simulink model "UAV_sync_unknown_gap_sim"  (R2018b)
settings: Solver=ode23tb  StartTime=0.0  StopTime=35  RelTol=1e-3
values from neighbouring files (symbols this model uses):
  Bm = [zeros(6,6); eye(6)]    [UAV_sync_unknown.m]    (also in UAV_sync_unknown_gap.m)
  C_rho = 1.225    [SC42120_UAV_Preconditions.m]
  D0 = [M0 0 0 0 0 0 ... (first row only)    [SC42120_UAV_Preconditions.m]
  Derivative_gain_phi = 50    [SC42120_UAV_Preconditions.m]
  Derivative_gain_psi = 50    [SC42120_UAV_Preconditions.m]
  Derivative_gain_theta = 50    [SC42120_UAV_Preconditions.m]
  Derivative_gain_x = 50    [SC42120_UAV_Preconditions.m]
  Derivative_gain_y = 50    [SC42120_UAV_Preconditions.m]
  Derivative_gain_z = 50    [SC42120_UAV_Preconditions.m]
  G = 9.80665    [SC42120_UAV_Preconditions.m]
  g0 = [0;0;-M0*G;0;0;0]    [SC42120_UAV_Preconditions.m]
  I0 = [0.02 0 -0.01 ... (first row only)    [SC42120_UAV_Preconditions.m]
  I2 = 2*[0.1 0 -0.01 ... (first row only)    [UAV_sync_known.m]    (also in UAV_sync_unknown.m; UAV_sync_unknown_gap.m)
  InitWind = [0;0;0]    [SC42120_UAV_Preconditions.m]
  Kp = diag(P)    [SC42120_UAV_Preconditions.m]
  Kv = diag(V)    [SC42120_UAV_Preconditions.m]
  M0 = 10    [SC42120_UAV_Preconditions.m]
  M1 = 20    [UAV_sync_known.m]    (also in UAV_sync_unknown.m; UAV_sync_unknown_gap.m)
  M2 = 30    [UAV_sync_known.m]    (also in UAV_sync_unknown.m; UAV_sync_unknown_gap.m)
  M3 = 40    [UAV_sync_known.m]    (also in UAV_sync_unknown.m; UAV_sync_unknown_gap.m)
  M4 = 50    [UAV_sync_known.m]    (also in UAV_sync_unknown.m; UAV_sync_unknown_gap.m)
  P = [Proportional_x Proportional_y Proportional_z Proportional_phi Proportional_theta Proportional_psi]    [SC42120_UAV_Preconditions.m]    (also in UAV_sync_unknown.m = lyap(Am',Q); UAV_sync_unknown_gap.m = lyap(Am',Q); drawDATCOMaircraft.m = temparray)
  Proportional_phi = 50    [SC42120_UAV_Preconditions.m]
  Proportional_psi = 50    [SC42120_UAV_Preconditions.m]
  Proportional_theta = 50    [SC42120_UAV_Preconditions.m]
  Proportional_x = 50    [SC42120_UAV_Preconditions.m]
  Proportional_y = 50    [SC42120_UAV_Preconditions.m]
  Proportional_z = 50    [SC42120_UAV_Preconditions.m]
  x_gap = 50    [UAV_sync_unknown_gap.m]
  y_gap = 100    [UAV_sync_unknown_gap.m]
undefined symbols (not defined in the file or in its folder): Aero, APlane, Bxl, C, Ctr, deg, DiscIntNeverNeededParam, F, Guid, Init, Light, MIL, Path, rad, s, Trim, Utility
libraries: aerolibconvert2 x37, sharedutil x20, simulink x15, dspsigops x7, shared6dof x6, aerolibasang x4, simulink_extras x3, aerolibadyn x1, aerolibtransform2 x1, aerolibwind2 x1
(part 1 of 7)
settings Model: Creator=kunal  LastModifiedBy=TUDelft SID
settings SolverCC: ZeroCrossAlgorithm=Adaptive

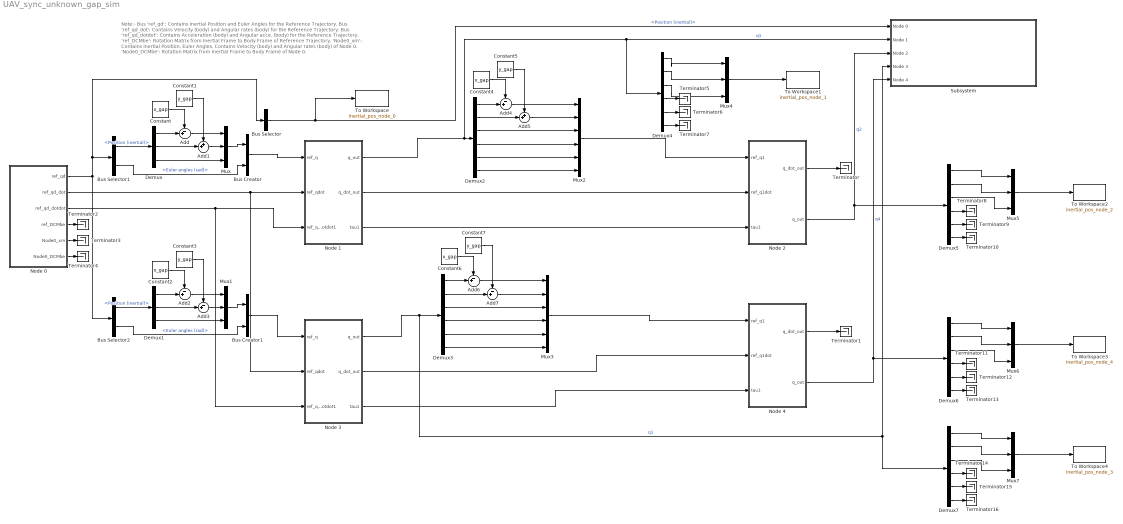
== system UAV_sync_unknown_gap_sim ==
  note: Note:-
      | Bus 'ref_qd': Contains Inertial Position and Euler Angles for the Reference Trajectory.
      | Bus 'ref_qd_dot': Contains Velocity (body) and Angular rates (body) for the Reference Trajectory.
      | Bus 'ref_qd_dotdot': Contains Acceleration (body) and Angular acce. (body) for the Reference Trajectory.
      | 'ref_DCMbe': Rotation Matrix from Inertial Frame to Body Frame of Reference Trajectory.
      | 'Node0_xm': Contains Inertial Position, Euler Angles, Contains Velocity (body) and Angular rates (body) of Node 0.
      | 'Node0_DCMbe': Rotation Matrix from Inertial Frame to Body Frame of Node 0.
  Add{,2..4,6..7} (6 alike) : Sum  Inputs=-+|
  Add1 : Sum  Inputs=++|
  Add5 : Sum  Inputs=++|
  Bus Creator : BusCreator  Inputs=2
  Bus Creator1 : BusCreator  Inputs=2
  Bus Selector : BusSelector  OutputSignals=Position (inertial)
  Bus Selector1 : BusSelector  OutputSignals=Position (inertial),Euler angles (rad)
  Bus Selector2 : BusSelector  OutputSignals=Position (inertial),Euler angles (rad)
  Constant{,2,4,6} (4 alike) : Constant  Value=x_gap
  Constant{1,3,5,7} (4 alike) : Constant  Value=y_gap
  Demux : Demux  Outputs=3
  Demux1 : Demux  Outputs=3
  Demux{2..7} (6 alike) : Demux  Outputs=6
  Mux{,1,4..7} (6 alike) : Mux  Inputs=3
  Mux2 : Mux  Inputs=6
  Mux3 : Mux  Inputs=6
  Node 0 : Subsystem
  Node 1 : Subsystem
  Node 2 : Subsystem
  Node 3 : Subsystem
  Node 4 : Subsystem
  Subsystem : Subsystem
  Terminator{,1..16} (17 alike) : Terminator
  To Workspace : ToWorkspace  VariableName=inertial_pos_node_0  SaveFormat=Timeseries  SampleTime=-1
  To Workspace1 : ToWorkspace  VariableName=inertial_pos_node_1  SaveFormat=Timeseries  SampleTime=-1
  To Workspace2 : ToWorkspace  VariableName=inertial_pos_node_2  SaveFormat=Timeseries  SampleTime=-1
  To Workspace3 : ToWorkspace  VariableName=inertial_pos_node_4  SaveFormat=Timeseries  SampleTime=-1
  To Workspace4 : ToWorkspace  VariableName=inertial_pos_node_3  SaveFormat=Timeseries  SampleTime=-1
  wires:
  Node 1/2(q_dot_out) -> Node 2/2(ref_q1dot)
  Node 0/3(ref_qd_dotdot) -> Node 3/3(ref_qd_dotdot1), Node 1/3(ref_qd_dotdot1)
  Node 0/2(ref_qd_dot) -> Node 3/2(ref_qdot), Node 1/2(ref_qdot)
  Node 1/3(tau1) -> Node 2/3(tau1)
  Node 0/1(ref_qd) -> Bus Selector1/1, Bus Selector/1, Bus Selector2/1
  Bus Selector/1 -> To Workspace/1, Subsystem/1("Node 0 ")  "<Position (inertial)>"
  Node 2/2(q_out) -> Subsystem/3(Node 2), Demux5/1  "q2"
  Node 4/2(q_out) -> Demux6/1, Subsystem/5(Node 4)  "q4"
  Node 2/1(q_dot_out) -> Terminator/1
  Node 4/1(q_dot_out) -> Terminator1/1
  Node 0/4(ref_DCMbe) -> Terminator2/1
  Node 0/5(Node0_xm) -> Terminator3/1
  Node 0/6(Node0_DCMbe) -> Terminator4/1
  Bus Selector1/1 -> Demux/1  "<Position (inertial)>"
  Demux/1 -> Add/2
  Constant/1 -> Add/1
  Demux/2 -> Add1/2
  Constant1/1 -> Add1/1
  Demux/3 -> Mux/3
  Add1/1 -> Mux/2
  Add/1 -> Mux/1
  Mux/1 -> Bus Creator/1
  Bus Selector1/2 -> Bus Creator/2  "<Euler angles (rad)>"
  Bus Creator/1 -> Node 1/1(ref_q)
  Mux1/1 -> Bus Creator1/1
  Add3/1 -> Mux1/2
  Demux1/1 -> Add2/2
  Bus Selector2/2 -> Bus Creator1/2  "<Euler angles (rad)>"
  Bus Selector2/1 -> Demux1/1  "<Position (inertial)>"
  Demux1/3 -> Mux1/3
  Demux1/2 -> Add3/2
  Constant3/1 -> Add3/1
  Add2/1 -> Mux1/1
  Constant2/1 -> Add2/1
  Bus Creator1/1 -> Node 3/1(ref_q)
  Node 1/1(q_out) -> Demux4/1, Subsystem/2(Node 1), Demux2/1  "q1"
  Demux2/1 -> Add4/2
  Demux2/2 -> Add5/2
  Constant5/1 -> Add5/1
  Constant4/1 -> Add4/1
  Add4/1 -> Mux2/1
  Add5/1 -> Mux2/2
  Demux2/3 -> Mux2/3
  Demux2/4 -> Mux2/4
  Demux2/5 -> Mux2/5
  Demux2/6 -> Mux2/6
  Mux2/1 -> Node 2/1(ref_q1)
  Add7/1 -> Mux3/2
  Demux3/3 -> Mux3/3
  Constant7/1 -> Add7/1
  Demux3/5 -> Mux3/5
  Constant6/1 -> Add6/1
  Add6/1 -> Mux3/1
  Demux3/6 -> Mux3/6
  Demux3/2 -> Add7/2
  Demux3/1 -> Add6/2
  Demux3/4 -> Mux3/4
  Node 3/1(q_out) -> Subsystem/4(Node 3), Demux7/1, Demux3/1  "q1"
  Mux3/1 -> Node 4/1(ref_q1)
  Node 3/2(q_dot_out) -> Node 4/2(ref_q1dot)
  Node 3/3(tau1) -> Node 4/3(tau1)
  Demux4/1 -> Mux4/1
  Demux4/2 -> Mux4/2
  Demux4/3 -> Mux4/3
  Mux4/1 -> To Workspace1/1
  Demux4/4 -> Terminator5/1
  Demux4/5 -> Terminator6/1
  Demux4/6 -> Terminator7/1
  Mux5/1 -> To Workspace2/1
  Demux5/6 -> Terminator10/1
  Demux5/4 -> Terminator8/1
  Demux5/5 -> Terminator9/1
  Demux5/1 -> Mux5/1
  Demux5/2 -> Mux5/2
  Demux5/3 -> Mux5/3
  Mux6/1 -> To Workspace3/1
  Demux6/6 -> Terminator13/1
  Demux6/4 -> Terminator11/1
  Demux6/5 -> Terminator12/1
  Demux6/1 -> Mux6/1
  Demux6/2 -> Mux6/2
  Demux6/3 -> Mux6/3
  Mux7/1 -> To Workspace4/1
  Demux7/6 -> Terminator16/1
  Demux7/4 -> Terminator14/1
  Demux7/5 -> Terminator15/1
  Demux7/1 -> Mux7/1
  Demux7/2 -> Mux7/2
  Demux7/3 -> Mux7/3

== system UAV_sync_unknown_gap_sim/Node 0 ==
  Bus Creator : BusCreator  Inputs=2
  Bus Creator1 : BusCreator  Inputs=2
  Bus Creator2 : BusCreator  Inputs=2
  Bus Creator3 : BusCreator  Inputs=4
  Bus Selector : BusSelector  OutputSignals=PlantData.Position (inertial),PlantData.Euler angles (rad),PlantData.Velocity (body),PlantData.Angular rates (body) (rad/s),PlantData.Accelerations (body/body),PlantData.Angular accelerations (body/body),PlantData.From inertial to body matrix
  Bus Selector1 : BusSelector  OutputSignals=Position (inertial),Euler angles (rad),Velocity (body),Angular rates (body),MatrixTransformation(Inertial-Body)
  Node 0 : Subsystem
  VF Approach : Subsystem
  ref_qd : Outport
  ref_qd_dot : Outport  Port=2
  ref_qd_dotdot : Outport  Port=3
  ref_DCMbe : Outport  Port=4
  Node0_xm : Outport  Port=5
  Node0_DCMbe : Outport  Port=6
  wires:
  VF Approach/1(VF_System_Parameters) -> Node 0/1(VF_System_Parameters)
  VF Approach/2(PlantData) -> Bus Selector/1
  Bus Selector/1 -> Bus Creator/1  "<Position (inertial)>"
  Bus Selector/2 -> Bus Creator/2  "<Euler angles (rad)>"
  Bus Creator/1 -> ref_qd/1
  Bus Selector/4 -> Bus Creator1/2  "<Angular rates (body) (rad/s)>"
  Bus Selector/3 -> Bus Creator1/1  "<Velocity (body)>"
  Bus Creator1/1 -> ref_qd_dot/1
  Bus Selector/6 -> Bus Creator2/2  "<Angular accelerations (body/body)>"
  Bus Selector/5 -> Bus Creator2/1  "<Accelerations (body/body)>"
  Bus Creator2/1 -> ref_qd_dotdot/1
  Bus Selector/7 -> ref_DCMbe/1  "<From inertial to body matrix>"
  Node 0/1(Node0_Data) -> Bus Selector1/1
  Bus Selector1/1 -> Bus Creator3/1  "<Position (inertial)>"
  Bus Selector1/3 -> Bus Creator3/3  "<Velocity (body)>"
  Bus Selector1/4 -> Bus Creator3/4  "<Angular rates (body)>"
  Bus Creator3/1 -> Node0_xm/1
  Bus Selector1/5 -> Node0_DCMbe/1  "<MatrixTransformation(Inertial-Body)>"
  Bus Selector1/2 -> Bus Creator3/2  "<Euler angles (rad)>"

== system UAV_sync_unknown_gap_sim/Node 1 ==
  ref_q : Inport
  ref_qdot : Inport  Port=2
  ref_qd_dotdot1 : Inport  Port=3
  Node 1 : Subsystem
  q_out : Outport
  q_dot_out : Outport  Port=2
  tau1 : Outport  Port=3
  wires:
  ref_q/1 -> Node 1/1(ref_q)
  ref_qdot/1 -> Node 1/2(ref_q_dot)
  ref_qd_dotdot1/1 -> Node 1/3(ref_q_dotdot)
  Node 1/1(q_dot_out) -> q_dot_out/1
  Node 1/2(q_out) -> q_out/1
  Node 1/3(tau1) -> tau1/1

== system UAV_sync_unknown_gap_sim/Node 2 ==
  ref_q1 : Inport
  ref_q1dot : Inport  Port=2
  tau1 : Inport  Port=3
  Node 2 : Subsystem
  q_dot_out : Outport
  q_out : Outport  Port=2
  wires:
  ref_q1/1 -> Node 2/1(ref_q)
  ref_q1dot/1 -> Node 2/2(ref_q_dot)
  Node 2/1(q_dot_out) -> q_dot_out/1
  Node 2/2(q_out) -> q_out/1
  tau1/1 -> Node 2/3(tau)

== system UAV_sync_unknown_gap_sim/Node 3 ==
  ref_q : Inport
  ref_qdot : Inport  Port=2
  ref_qd_dotdot1 : Inport  Port=3
  Node 1 : Subsystem
  q_out : Outport
  q_dot_out : Outport  Port=2
  tau1 : Outport  Port=3
  wires:
  ref_q/1 -> Node 1/1(ref_q)
  ref_qdot/1 -> Node 1/2(ref_q_dot)
  ref_qd_dotdot1/1 -> Node 1/3(ref_q_dotdot)
  Node 1/1(q_dot_out) -> q_dot_out/1
  Node 1/2(q_out) -> q_out/1
  Node 1/3(tau1) -> tau1/1

== system UAV_sync_unknown_gap_sim/Node 4 ==
  ref_q1 : Inport
  ref_q1dot : Inport  Port=2
  tau1 : Inport  Port=3
  Node 2 : Subsystem
  q_dot_out : Outport
  q_out : Outport  Port=2
  wires:
  ref_q1/1 -> Node 2/1(ref_q)
  ref_q1dot/1 -> Node 2/2(ref_q_dot)
  Node 2/1(q_dot_out) -> q_dot_out/1
  Node 2/2(q_out) -> q_out/1
  tau1/1 -> Node 2/3(tau)

== system UAV_sync_unknown_gap_sim/Subsystem ==
  "Node 0 " : Inport
  Node 1 : Inport  Port=2
  Node 2 : Inport  Port=3
  Node 3 : Inport  Port=4
  Node 4 : Inport  Port=5
  Demux : Demux  Outputs=3
  Demux{1..3,6} (4 alike) : Demux  Outputs=6
  Gain{,1..4} (5 alike) : Gain  Gain=-1
  Scope X : Scope  NumInputPorts=5
  Scope Y : Scope  NumInputPorts=5
  Scope Z : Scope  NumInputPorts=5
  Terminator{,1..11} (12 alike) : Terminator
  wires:
  Demux6/3 -> Gain1/1  "Node 1"
  Demux6/6 -> Terminator2/1
  Gain1/1 -> Scope Z/2  "Node 1"
  Demux6/1 -> Scope X/2  "Node 1"
  Demux6/4 -> Terminator/1
  Demux6/5 -> Terminator1/1
  Demux/3 -> Gain/1  "Node 0"
  Demux6/2 -> Scope Y/2  "Node 1"
  Gain/1 -> Scope Z/1  "Node 0"
  Node 1/1 -> Demux6/1
  Demux/2 -> Scope Y/1  "Node 0"
  Demux1/5 -> Terminator4/1
  Demux1/4 -> Terminator3/1
  Demux1/6 -> Terminator5/1
  Node 2/1 -> Demux1/1
  Demux1/1 -> Scope X/3  "Node 2"
  Demux1/3 -> Gain2/1  "Node 2"
  Gain2/1 -> Scope Z/3  "Node 2"
  Demux1/2 -> Scope Y/3  "Node 2"
  Demux2/6 -> Terminator8/1
  Demux2/4 -> Terminator6/1
  Demux2/5 -> Terminator7/1
  Node 3/1 -> Demux2/1
  Demux2/1 -> Scope X/4  "Node 3"
  Demux2/3 -> Gain3/1  "Node 3"
  Demux2/2 -> Scope Y/4  "Node 3"
  Gain3/1 -> Scope Z/4  "Node 3"
  Demux3/6 -> Terminator11/1
  Demux3/4 -> Terminator9/1
  Demux3/5 -> Terminator10/1
  Node 4/1 -> Demux3/1
  Demux3/1 -> Scope X/5  "Node 4"
  Demux3/2 -> Scope Y/5  "Node 4"
  Demux3/3 -> Gain4/1  "Node 4"
  Gain4/1 -> Scope Z/5  "Node 3"
  "Node 0 "/1 -> Demux/1
  Demux/1 -> Scope X/1  "Node 0"

== system UAV_sync_unknown_gap_sim/Node 0/Node 0 ==
  note: Inverse Dynamics
  VF_System_Parameters : Inport
  6DOF (Euler Angles) : shared6dof/6DOF (Euler Angles)  units=Metric (MKS)  mtype=Fixed  rep=Euler Angles  xme_0=init_pos0  Vm_0=init_vel0  eul_0=init_eul0  pm_0=init_ang0  mass_0=M0  mass_e=0.5  mass_f=2.0  inertia=I0  inertia_e=eye(3)  inertia_f=2*eye(3)  k_quat=1.0  vre_flag=on  abi_flag=off  aMode=aMode  xme_statename=''  Vm_statename=''  eul_statename=''  quat_statename=''  pm_statename=''  mass_statename=''
      settings: SourceProductBaseCode=AE
  ALL_DATA2 : Goto  Commented=on  GotoTag=DERIVED_DATA
  Add : Sum
  Bus Creator : BusCreator  Inputs=10
  Constant8 : Constant  Value=M0*G
  Demux5 : Demux  Outputs=6
  Derived Data : Subsystem
  Gain : Gain  Gain=[1 1 -1]
  Inverse Dynamics Control : Subsystem
  Mux8 : Mux  Inputs=3
  Mux9 : Mux  Inputs=3
  Product : Product  Multiplication=Matrix(*)
  Subsystem : Subsystem
  Wind : Subsystem
  tau : Sum  Inputs=+++
  Node0_Data : Outport
  wires:
  Gain/1 -> Product/2, Bus Creator/3  "xyh"
  6DOF (Euler Angles)/1 -> Bus Creator/1  "Velocity (inertial)"
  Mux8/1 -> 6DOF (Euler Angles)/1
  6DOF (Euler Angles)/3 -> Bus Creator/4  "Euler angles (rad)"
  Bus Creator/1 -> [AIRCRAFT_DATA]
  6DOF (Euler Angles)/6 -> Bus Creator/7  "Angular rates (body)"
  6DOF (Euler Angles)/8 -> Bus Creator/9  "Acceleration (Body)"
  Mux9/1 -> 6DOF (Euler Angles)/2
  6DOF (Euler Angles)/7 -> Bus Creator/8  "Angular accelerations (body)"
  6DOF (Euler Angles)/5 -> Bus Creator/6  "Velocity (body)"
  6DOF (Euler Angles)/2 -> Gain/1, Bus Creator/2  "Position (inertial)"
  6DOF (Euler Angles)/4 -> Product/1, Bus Creator/5  "MatrixTransformation(Inertial-Body)"
  tau/1 -> Demux5/1
  Demux5/2 -> Mux8/2
  Demux5/4 -> Mux9/1
  Demux5/5 -> Mux9/2
  Demux5/6 -> Mux9/3
  [WIND_DATA] -> Derived Data/1(In1)
  [AIRCRAFT_DATA] -> Derived Data/2(In2)
  Derived Data/1(Derived_Condition) -> ALL_DATA2/1
  [AIRCRAFT_DATA] -> Wind/1(In1)
  Wind/1(Out1) -> [WIND_DATA]
  Inverse Dynamics Control/1(D_qddot) -> tau/1
  Inverse Dynamics Control/2(C_qdot) -> tau/2
  Inverse Dynamics Control/3(g(q)) -> tau/3
  Constant8/1 -> Add/2
  Demux5/3 -> Add/1
  Add/1 -> Mux8/3
  Demux5/1 -> Mux8/1
  [AIRCRAFT_DATA] -> Inverse Dynamics Control/2(Aircraft Data), Node0_Data/1
  VF_System_Parameters/1 -> Subsystem/1(VF_System_Parameters)
  Subsystem/1(References) -> Inverse Dynamics Control/1(References)
  Product/1 -> Bus Creator/10  "xyh_body"

== system UAV_sync_unknown_gap_sim/Node 0/VF Approach ==
  note: Created by: Stefano Farì
      | Last edit: Mar 2018
  note: Fixed-wing UAV Simulator
  note: Ground Hit
  note: Wind
  note: To workspace
  note: MAIN
  AUTOPILOT : Subsystem
  BIXLER DYNAMICS : Subsystem
  Bus Selector3 : BusSelector  OutputSignals=PlantData.xyh_body,PlantData.Euler angles (rad),PlantData.Velocity (body),PlantData.Angular rates (body) (rad/s),PlantData.Accelerations (body/body),PlantData.Angular accelerations (body/body)
  ENVIRONMENT : Subsystem
  GROUND HIT : Subsystem
  MANUAL INPUTS : Subsystem
  Mux : Mux  Inputs=6
  PATH FOLLOWING : Subsystem
  PATH MANAGER : Subsystem
  TO WORKSPACE : Subsystem
  VF_System_Parameters : Outport
  PlantData : Outport  Port=2
  wires:
  MANUAL INPUTS/2(EnvData.) -> BIXLER DYNAMICS/2(EnvData)
  [PlantData] -> PATH MANAGER/1(PlantData)
  MANUAL INPUTS/4(VF.) -> BIXLER DYNAMICS/4(VF)
  [VF] -> TO WORKSPACE/4(VF)
  MANUAL INPUTS/3(GuidData.) -> BIXLER DYNAMICS/3(GuidData)
  [EnvData] -> PATH MANAGER/3(EnvData)
  [PlantData] -> PlantData/1, Bus Selector3/1
  BIXLER DYNAMICS/4(GuidData.) -> [GuidData]
  MANUAL INPUTS/1(CtrBus.) -> BIXLER DYNAMICS/1(ControlActions)
  AUTOPILOT/3(VF.) -> MANUAL INPUTS/3(VF)
  PATH MANAGER/2(DerCond.) -> PATH FOLLOWING/2(DerCond)
  PATH FOLLOWING/1("PlantData. ") -> AUTOPILOT/1(PlantData)
  AUTOPILOT/4(GuidData.) -> MANUAL INPUTS/4(GuidData)
  [GuidData] -> TO WORKSPACE/5(GuidData)
  [DerCond] -> TO WORKSPACE/2(DerCond)
  PATH FOLLOWING/5(GuidData.) -> AUTOPILOT/5(GuidData)
  BIXLER DYNAMICS/5(VF.) -> [VF]
  PATH FOLLOWING/2("DerCond. ") -> AUTOPILOT/2(DerCond)
  BIXLER DYNAMICS/1(PlantData.) -> [PlantData]
  [PlantData] -> GROUND HIT/1(PlantData)
  [PlantData] -> ENVIRONMENT/1(PlantData)
  BIXLER DYNAMICS/3(ControlBus.) -> [ControlBus]
  AUTOPILOT/2(EnvData.) -> MANUAL INPUTS/2(EnvData)
  PATH MANAGER/1(Plantdata.) -> PATH FOLLOWING/1(PlantData)
  PATH MANAGER/4(GuidData.) -> PATH FOLLOWING/4(GuidData)
  ENVIRONMENT/1(EnvData) -> [EnvData]
  PATH FOLLOWING/4(VF.) -> AUTOPILOT/4(VF)
  Bus Selector3/4 -> Mux/4  "<Angular rates (body) (rad/s)>"
  PATH MANAGER/3(EnvData.) -> PATH FOLLOWING/3(EnvData)
  [PlantData] -> TO WORKSPACE/1(PlantData)
  [DerCond] -> PATH MANAGER/2(DerCond)
  BIXLER DYNAMICS/2(DerCond.) -> [DerCond]
  [EnvData] -> TO WORKSPACE/6(EnvData)
  [ControlBus] -> TO WORKSPACE/3(ControlBus)
  AUTOPILOT/1(CtrBus.) -> MANUAL INPUTS/1(CtrBus)
  PATH FOLLOWING/3(EnvData.) -> AUTOPILOT/3(EnvData)
  Mux/1 -> VF_System_Parameters/1
  Bus Selector3/1 -> Mux/1  "<xyh_body>"
  Bus Selector3/2 -> Mux/2  "<Euler angles (rad)>"
  Bus Selector3/3 -> Mux/3  "<Velocity (body)>"
  Bus Selector3/5 -> Mux/5  "<Accelerations (body/body)>"
  Bus Selector3/6 -> Mux/6  "<Angular accelerations (body/body)>"

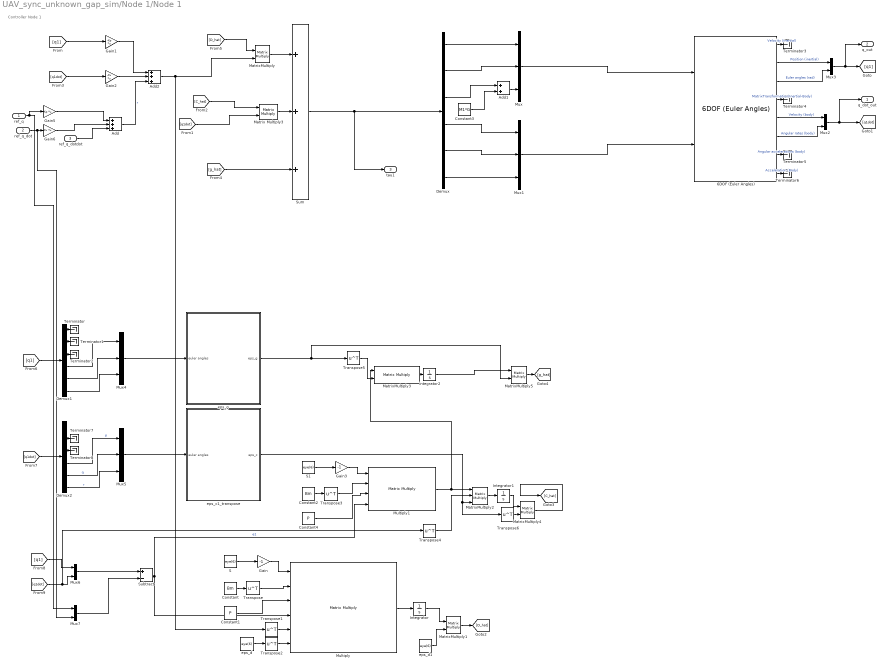
== system UAV_sync_unknown_gap_sim/Node 1/Node 1 ==
  note: Controller Node 1
  ref_q : Inport
  ref_q_dot : Inport  Port=2
  ref_q_dotdot : Inport  Port=3
  6DOF (Euler Angles) : shared6dof/6DOF (Euler Angles)  units=Metric (MKS)  mtype=Fixed  rep=Euler Angles  xme_0=init_pos1  Vm_0=init_vel1  eul_0=init_eul1  pm_0=init_ang1  mass_0=M1  mass_e=0.5  mass_f=2.0  inertia=I1  inertia_e=eye(3)  inertia_f=2*eye(3)  k_quat=1.0  vre_flag=on  abi_flag=off  aMode=aMode  xme_statename=''  Vm_statename=''  eul_statename=''  quat_statename=''  pm_statename=''  mass_statename=''
      settings: SourceProductBaseCode=AE
  Add : Sum  Inputs=+++
  Add1 : Sum
  Add2 : Sum  Inputs=3
  Constant : Constant  Value=Bm
  Constant1 : Constant  Value=P
  Constant2 : Constant  Value=Bm
  Constant3 : Constant  Value=M1*G
  Constant4 : Constant  Value=P
  Demux : Demux  Outputs=6
  Demux1 : Demux  Outputs=6
  Demux2 : Demux  Outputs=6
  Gain : Gain  Gain=-1
  Gain1 : Gain  Gain=-Kp  Multiplication=Matrix(K*u)
  Gain2 : Gain  Gain=-Kv  Multiplication=Matrix(K*u)
  Gain3 : Gain  Gain=-1
  Gain5 : Gain  Gain=Kp  Multiplication=Matrix(K*u)
  Gain6 : Gain  Gain=Kv  Multiplication=Matrix(K*u)
  Integrator : Integrator
  Integrator1 : Integrator
  Integrator2 : Integrator
  Matrix Multiply3 : Product  Multiplication=Matrix(*)
  MatrixMultiply{,1,3..5} (5 alike) : Product  Multiplication=Matrix(*)
  MatrixMultiply2 : Product  Inputs=3  Multiplication=Matrix(*)
  Multiply : Product  Inputs=6  Multiplication=Matrix(*)
  Multiply1 : Product  Inputs=4  Multiplication=Matrix(*)
  Mux{,1,4..5} (4 alike) : Mux  Inputs=3
  Mux{2..3,6..7} (4 alike) : Mux  Inputs=2
  S : Constant  Value=eye(6)
  S1 : Constant  Value=eye(6)
  Subtract : Sum  Inputs=+-
  Sum : Sum  Inputs=+++
  Terminator{,1..8} (9 alike) : Terminator
  Transpose{,1..6} (7 alike) : Math  Operator=transpose  SaturateOnIntegerOverflow=on
  eps_c1_transpose : Subsystem
  eps_d : Constant  Value=eye(6)
  eps_d1 : Constant  Value=eye(6)
  eps_g : Subsystem
  q_dot_out : Outport
  q_out : Outport  Port=2
  tau1 : Outport  Port=3
  wires:
  6DOF (Euler Angles)/3 -> Mux3/2  "Euler angles (rad)"
  6DOF (Euler Angles)/6 -> Mux2/2  "Angular rates (body)"
  6DOF (Euler Angles)/5 -> Mux2/1  "Velocity (body)"
  6DOF (Euler Angles)/2 -> Mux3/1  "Position (inertial)"
  ref_q_dotdot/1 -> Add/3
  ref_q_dot/1 -> Mux7/2, Gain6/1
  [q1] -> Gain1/1
  [q1dot] -> Matrix Multiply3/2
  Sum/1 -> tau1/1, Demux/1
  Demux/1 -> Mux/1
  Demux/2 -> Mux/2
  Demux/6 -> Mux1/3
  Demux/5 -> Mux1/2
  Demux/4 -> Mux1/1
  Mux/1 -> 6DOF (Euler Angles)/1
  Mux1/1 -> 6DOF (Euler Angles)/2
  Mux2/1 -> q_dot_out/1, [q1dot]
  Gain5/1 -> Add/1
  Gain6/1 -> Add/2
  Add1/1 -> Mux/3
  Demux/3 -> Add1/1
  Constant3/1 -> Add1/2
  6DOF (Euler Angles)/1 -> Terminator3/1  "Velocity (inertial)"
  6DOF (Euler Angles)/4 -> Terminator4/1  "MatrixTransformation(Inertial-Body)"
  6DOF (Euler Angles)/7 -> Terminator5/1  "Angular accelerations (body)"
  6DOF (Euler Angles)/8 -> Terminator6/1  "Acceleration (Body)"
  Mux3/1 -> q_out/1, [q1]
  [q1dot] -> Gain2/1
  [C_hat] -> Matrix Multiply3/1
  [g_hat] -> Sum/3
  Matrix Multiply3/1 -> Sum/2
  Gain2/1 -> Add2/2
  Add/1 -> Add2/3  "r"
  Gain1/1 -> Add2/1
  MatrixMultiply/1 -> Sum/1
  Add2/1 -> Transpose1/1, MatrixMultiply/2
  [D_hat] -> MatrixMultiply/1
  Demux1/5 -> Mux4/2
  [q1] -> Demux1/1
  Demux1/1 -> Terminator/1
  Demux1/6 -> Mux4/3
  Demux1/4 -> Mux4/1
  Mux4/1 -> eps_g/1(euler angles)
  Demux1/2 -> Terminator1/1
  Demux1/3 -> Terminator2/1
  Demux2/6 -> Mux5/3  "r"
  [q1dot] -> Demux2/1
  Demux2/4 -> Mux5/1  "p"
  Demux2/3 -> Terminator8/1
  Mux5/1 -> eps_c1_transpose/1(euler angles)
  Demux2/5 -> Mux5/2  "q"
  Demux2/2 -> Terminator7/1
  [q1] -> Mux6/1
  [q1dot] -> Transpose4/1, Mux6/2
  Mux6/1 -> Subtract/1
  Mux7/1 -> Subtract/2
  Gain/1 -> Multiply/1
  S/1 -> Gain/1
  Constant/1 -> Transpose/1
  Transpose/1 -> Multiply/2
  Multiply/1 -> Integrator/1
  Constant1/1 -> Multiply/3
  Subtract/1 -> Multiply/4, Multiply1/4  "e1"
  ref_q/1 -> Gain5/1, Mux7/1
  Transpose1/1 -> Multiply/5
  Transpose2/1 -> Multiply/6
  eps_d/1 -> Transpose2/1
  Integrator/1 -> MatrixMultiply1/1
  eps_d1/1 -> MatrixMultiply1/2
  MatrixMultiply1/1 -> [D_hat]
  Transpose3/1 -> Multiply1/2
  S1/1 -> Gain3/1
  Gain3/1 -> Multiply1/1
  Constant2/1 -> Transpose3/1
  Constant4/1 -> Multiply1/3
  Multiply1/1 -> MatrixMultiply3/1, MatrixMultiply2/1
  Transpose4/1 -> MatrixMultiply2/2
  eps_c1_transpose/1(eps_c) -> Transpose6/1, MatrixMultiply2/3
  MatrixMultiply2/1 -> Integrator1/1
  Transpose5/1 -> MatrixMultiply3/2
  eps_g/1(eps_g) -> MatrixMultiply5/2, Transpose5/1
  Integrator1/1 -> MatrixMultiply4/1
  MatrixMultiply4/1 -> [C_hat]
  MatrixMultiply3/1 -> Integrator2/1
  MatrixMultiply5/1 -> [g_hat]
  Integrator2/1 -> MatrixMultiply5/1
  Transpose6/1 -> MatrixMultiply4/2

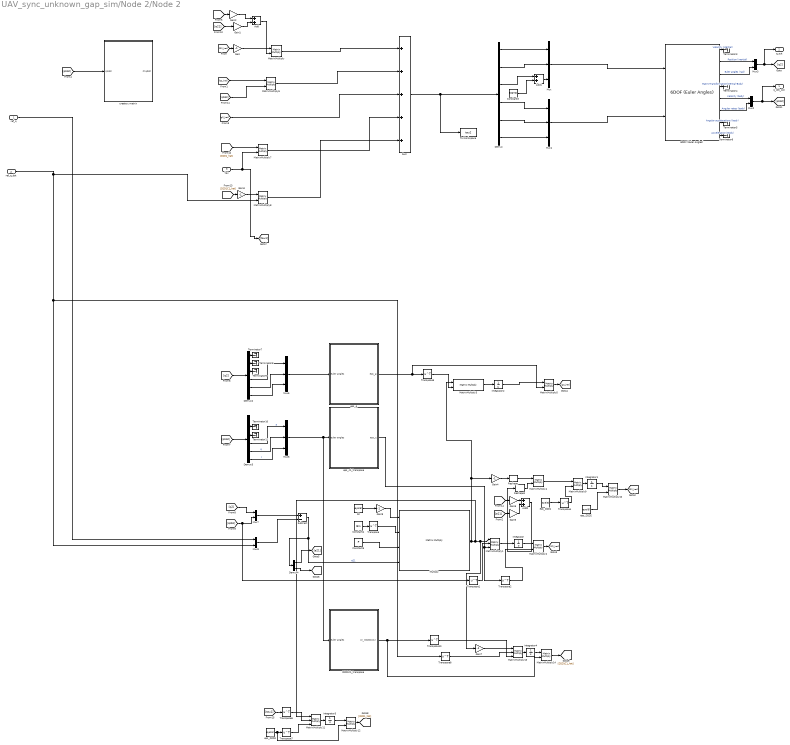
== system UAV_sync_unknown_gap_sim/Node 2/Node 2 ==
  ref_q : Inport
  ref_q_dot : Inport  Port=2
  tau : Inport  Port=3
  6DOF (Euler Angles) : shared6dof/6DOF (Euler Angles)  units=Metric (MKS)  mtype=Fixed  rep=Euler Angles  xme_0=init_pos2  Vm_0=init_vel2  eul_0=init_eul2  pm_0=init_ang2  mass_0=M2  mass_e=0.5  mass_f=2.0  inertia=I2  inertia_e=eye(3)  inertia_f=2*eye(3)  k_quat=1.0  vre_flag=on  abi_flag=off  aMode=aMode  xme_statename=''  Vm_statename=''  eul_statename=''  quat_statename=''  pm_statename=''  mass_statename=''
      settings: SourceProductBaseCode=AE
  Add : Sum
  Add1 : Sum
  Add2 : Sum
  Constant3 : Constant  Value=M2*G
  Constant4 : Constant  Value=Bm
  Constant5 : Constant  Value=P
  D2D1C1_transpose : Subsystem
  Demux : Demux  Outputs=6
  Demux2 : Demux  Outputs=6
  Demux3 : Demux  Outputs=6
  Demux4 : Demux  Outputs=2
  Gain{,3..4,7,9} (5 alike) : Gain  Gain=-1
  Gain1 : Gain  Gain=Kp  Multiplication=Matrix(K*u)
  Gain2 : Gain  Gain=Kv  Multiplication=Matrix(K*u)
  Gain5 : Gain  Gain=Kp  Multiplication=Matrix(K*u)
  Gain6 : Gain  Gain=Kv  Multiplication=Matrix(K*u)
  Integrator{,1..4} (5 alike) : Integrator
  MatrixMultiply{,2..10,12,14} (12 alike) : Product  Multiplication=Matrix(*)
  MatrixMultiply1 : Product  Inputs=3  Multiplication=Matrix(*)
  MatrixMultiply11 : Product  Inputs=3  Multiplication=Matrix(*)
  MatrixMultiply13 : Product  Inputs=3  Multiplication=Matrix(*)
  Multiply : Product  Inputs=4  Multiplication=Matrix(*)
  Mux{,1,5..6} (4 alike) : Mux  Inputs=3
  Mux{2..3,7..8} (4 alike) : Mux  Inputs=2
  Reshape : Reshape  OutputDimensionality=Column vector (2-D)
  Reshape1 : Reshape  OutputDimensionality=Row vector (2-D)
  S2 : Constant  Value=eye(6)
  Subtract : Sum  Inputs=+-
  Sum : Sum  Inputs=+++++
  Terminator{3..11} (9 alike) : Terminator
  To Workspace : ToWorkspace  VariableName=tau2  SaveFormat=Timeseries  SampleTime=-1
  Transpose{,1..2,4..8,10} (9 alike) : Math  Operator=transpose  SaturateOnIntegerOverflow=on
  create c matrix : Subsystem
  eps_D2D1 : Constant  Value=eye(6)
  eps_D2D2 : Constant  Value=eye(6)
  eps_D2D3 : Constant  Value=eye(6)
  eps_c1_transpose : Subsystem
  eps_g : Subsystem
  q_dot_out : Outport
  q_out : Outport  Port=2
  wires:
  6DOF (Euler Angles)/3 -> Mux3/2  "Euler angles (rad)"
  6DOF (Euler Angles)/6 -> Mux2/2  "Angular rates (body)"
  6DOF (Euler Angles)/5 -> Mux2/1  "Velocity (body)"
  6DOF (Euler Angles)/2 -> Mux3/1  "Position (inertial)"
  ref_q/1 -> Mux8/1
  ref_q_dot/1 -> MatrixMultiply8/2, Transpose8/1, Mux8/2
  Sum/1 -> To Workspace/1, Demux/1
  Demux/1 -> Mux/1
  Demux/2 -> Mux/2
  Demux/6 -> Mux1/3
  Demux/5 -> Mux1/2
  Demux/4 -> Mux1/1
  Mux/1 -> 6DOF (Euler Angles)/1
  Mux1/1 -> 6DOF (Euler Angles)/2
  Mux2/1 -> q_dot_out/1, [q2dot]
  Add1/1 -> Mux/3
  Demux/3 -> Add1/1
  Constant3/1 -> Add1/2
  [q2dot] -> create c matrix/1("q1dot ")
  6DOF (Euler Angles)/1 -> Terminator3/1  "Velocity (inertial)"
  6DOF (Euler Angles)/4 -> Terminator4/1  "MatrixTransformation(Inertial-Body)"
  6DOF (Euler Angles)/7 -> Terminator5/1  "Angular accelerations (body)"
  6DOF (Euler Angles)/8 -> Terminator6/1  "Acceleration (Body)"
  Mux3/1 -> q_out/1, [q2]
  Demux2/6 -> Mux5/3
  Demux2/1 -> Terminator7/1
  Mux6/1 -> D2D1C1_transpose/1(euler angles), eps_c1_transpose/1(euler angles)
  Demux3/4 -> Mux6/1  "p"
  Demux3/6 -> Mux6/3  "r"
  Demux3/2 -> Terminator10/1
  Demux3/3 -> Terminator11/1
  Constant5/1 -> Multiply/3
  Subtract/1 -> Demux4/1, Multiply/4  "e21"
  Integrator2/1 -> MatrixMultiply5/1
  Demux2/5 -> Mux5/2
  MatrixMultiply10/1 -> [D2_hat]
  Demux3/5 -> Mux6/2  "q"
  Constant4/1 -> Transpose/1
  [q2] -> Mux7/1
  [q2dot] -> Transpose1/1, Mux7/2
  Transpose/1 -> Multiply/2
  S2/1 -> Gain9/1
  MatrixMultiply3/1 -> Integrator2/1
  MatrixMultiply5/1 -> [g2_hat]
  Mux5/1 -> eps_g/1(euler angles)
  Demux2/4 -> Mux5/1
  Demux2/3 -> Terminator9/1
  Demux2/2 -> Terminator8/1
  eps_c1_transpose/1(eps_c) -> Transpose2/1, MatrixMultiply1/3
  Gain9/1 -> Multiply/1
  Transpose5/1 -> MatrixMultiply3/2
  eps_g/1(eps_g) -> MatrixMultiply5/2, Transpose5/1
  [q2dot] -> Demux3/1
  [q2] -> Demux2/1
  Mux8/1 -> Subtract/2
  Mux7/1 -> Subtract/1
  [D2_hat] -> Gain/1
  Demux4/2 -> [e21_dot]
  Demux4/1 -> [e21]
  [e21] -> Gain1/1
  [e21_dot] -> Gain2/1
  Gain1/1 -> Add/2
  Gain2/1 -> Add/1
  Gain/1 -> MatrixMultiply/1
  Add/1 -> MatrixMultiply/2
  MatrixMultiply/1 -> Sum/1
  [C2_hat] -> MatrixMultiply6/1
  [q2dot] -> MatrixMultiply6/2
  MatrixMultiply6/1 -> Sum/2
  [g2_hat] -> Sum/3
  [D2D1_hat] -> MatrixMultiply7/1
  tau/1 -> [tau1], MatrixMultiply7/2
  MatrixMultiply7/1 -> Sum/4
  [D2D1C1_hat] -> Gain3/1
  Gain3/1 -> MatrixMultiply8/1
  MatrixMultiply8/1 -> Sum/5
  Transpose1/1 -> MatrixMultiply1/2
  MatrixMultiply2/1 -> [C2_hat]
  MatrixMultiply1/1 -> Integrator/1
  Transpose2/1 -> MatrixMultiply2/2
  Multiply/1 -> MatrixMultiply3/1, Gain4/1, MatrixMultiply11/1, Gain7/1, MatrixMultiply1/1
  Integrator/1 -> MatrixMultiply2/1
  [e21] -> Gain5/1
  [e21_dot] -> Gain6/1
  Gain6/1 -> Add2/1
  Gain5/1 -> Add2/2
  eps_D2D1/1 -> Transpose4/1
  MatrixMultiply4/1 -> MatrixMultiply9/1
  Transpose4/1 -> MatrixMultiply9/2
  MatrixMultiply9/1 -> Integrator1/1
  eps_D2D2/1 -> MatrixMultiply10/2
  [tau1] -> Transpose6/1
  Transpose6/1 -> MatrixMultiply11/2
  eps_D2D3/1 -> MatrixMultiply12/2, Transpose7/1
  Transpose7/1 -> MatrixMultiply11/3
  MatrixMultiply11/1 -> Integrator3/1
  Integrator3/1 -> MatrixMultiply12/1
  MatrixMultiply12/1 -> [D2D1_hat]
  Gain7/1 -> MatrixMultiply13/1
  Transpose8/1 -> MatrixMultiply13/2
  MatrixMultiply13/1 -> Integrator4/1
  Integrator4/1 -> MatrixMultiply14/1
  D2D1C1_transpose/1("\\xi_{D2D1C1}") -> MatrixMultiply14/2, Transpose10/1
  MatrixMultiply14/1 -> [D2D1C1_hat]
  Transpose10/1 -> MatrixMultiply13/3
  Integrator1/1 -> MatrixMultiply10/1
  Gain4/1 -> Reshape/1
  Add2/1 -> Reshape1/1
  Reshape1/1 -> MatrixMultiply4/2
  Reshape/1 -> MatrixMultiply4/1

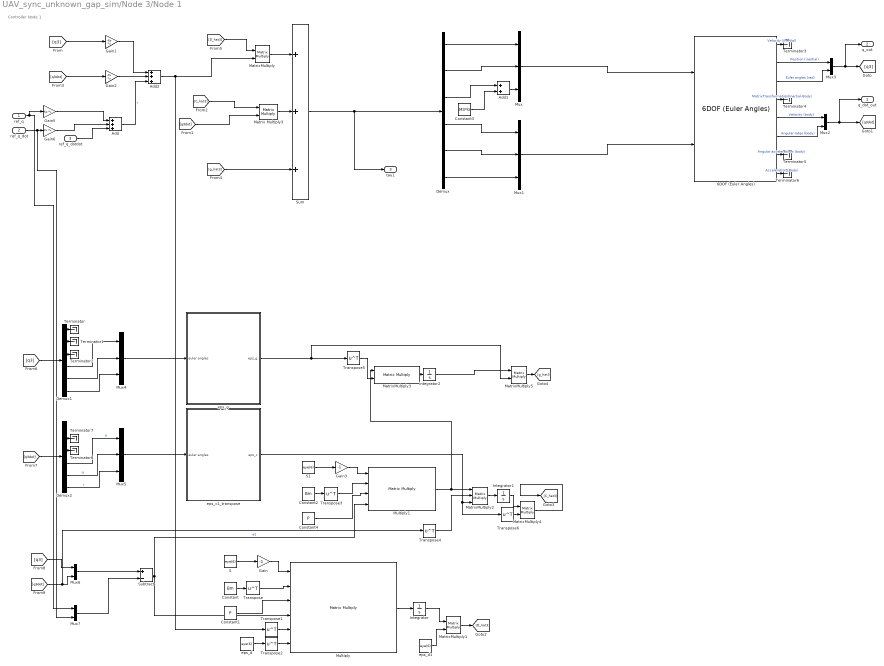
== system UAV_sync_unknown_gap_sim/Node 3/Node 1 ==
  note: Controller Node 1
  ref_q : Inport
  ref_q_dot : Inport  Port=2
  ref_q_dotdot : Inport  Port=3
  6DOF (Euler Angles) : shared6dof/6DOF (Euler Angles)  units=Metric (MKS)  mtype=Fixed  rep=Euler Angles  xme_0=init_pos3  Vm_0=init_vel3  eul_0=init_eul3  pm_0=init_ang3  mass_0=M3  mass_e=0.5  mass_f=2.0  inertia=I3  inertia_e=eye(3)  inertia_f=2*eye(3)  k_quat=1.0  vre_flag=on  abi_flag=off  aMode=aMode  xme_statename=''  Vm_statename=''  eul_statename=''  quat_statename=''  pm_statename=''  mass_statename=''
      settings: SourceProductBaseCode=AE
  Add : Sum  Inputs=+++
  Add1 : Sum
  Add2 : Sum  Inputs=3
  Constant : Constant  Value=Bm
  Constant1 : Constant  Value=P
  Constant2 : Constant  Value=Bm
  Constant3 : Constant  Value=M3*G
  Constant4 : Constant  Value=P
  Demux : Demux  Outputs=6
  Demux1 : Demux  Outputs=6
  Demux2 : Demux  Outputs=6
  Gain : Gain  Gain=-1
  Gain1 : Gain  Gain=-Kp  Multiplication=Matrix(K*u)
  Gain2 : Gain  Gain=-Kv  Multiplication=Matrix(K*u)
  Gain3 : Gain  Gain=-1
  Gain5 : Gain  Gain=Kp  Multiplication=Matrix(K*u)
  Gain6 : Gain  Gain=Kv  Multiplication=Matrix(K*u)
  Integrator : Integrator
  Integrator1 : Integrator
  Integrator2 : Integrator
  Matrix Multiply3 : Product  Multiplication=Matrix(*)
  MatrixMultiply{,1,3..5} (5 alike) : Product  Multiplication=Matrix(*)
  MatrixMultiply2 : Product  Inputs=3  Multiplication=Matrix(*)
  Multiply : Product  Inputs=6  Multiplication=Matrix(*)
  Multiply1 : Product  Inputs=4  Multiplication=Matrix(*)
  Mux{,1,4..5} (4 alike) : Mux  Inputs=3
  Mux{2..3,6..7} (4 alike) : Mux  Inputs=2
  S : Constant  Value=eye(6)
  S1 : Constant  Value=eye(6)
  Subtract : Sum  Inputs=+-
  Sum : Sum  Inputs=+++
  Terminator{,1..8} (9 alike) : Terminator
  Transpose{,1..6} (7 alike) : Math  Operator=transpose  SaturateOnIntegerOverflow=on
  eps_c1_transpose : Subsystem
  eps_d : Constant  Value=eye(6)
  eps_d1 : Constant  Value=eye(6)
  eps_g : Subsystem
  q_dot_out : Outport
  q_out : Outport  Port=2
  tau1 : Outport  Port=3
  wires:
  6DOF (Euler Angles)/3 -> Mux3/2  "Euler angles (rad)"
  6DOF (Euler Angles)/6 -> Mux2/2  "Angular rates (body)"
  6DOF (Euler Angles)/5 -> Mux2/1  "Velocity (body)"
  6DOF (Euler Angles)/2 -> Mux3/1  "Position (inertial)"
  ref_q_dotdot/1 -> Add/3
  ref_q_dot/1 -> Mux7/2, Gain6/1
  [q3] -> Gain1/1
  [q3dot] -> Matrix Multiply3/2
  Sum/1 -> tau1/1, Demux/1
  Demux/1 -> Mux/1
  Demux/2 -> Mux/2
  Demux/6 -> Mux1/3
  Demux/5 -> Mux1/2
  Demux/4 -> Mux1/1
  Mux/1 -> 6DOF (Euler Angles)/1
  Mux1/1 -> 6DOF (Euler Angles)/2
  Mux2/1 -> q_dot_out/1, [q3dot]
  Gain5/1 -> Add/1
  Gain6/1 -> Add/2
  Add1/1 -> Mux/3
  Demux/3 -> Add1/1
  Constant3/1 -> Add1/2
  6DOF (Euler Angles)/1 -> Terminator3/1  "Velocity (inertial)"
  6DOF (Euler Angles)/4 -> Terminator4/1  "MatrixTransformation(Inertial-Body)"
  6DOF (Euler Angles)/7 -> Terminator5/1  "Angular accelerations (body)"
  6DOF (Euler Angles)/8 -> Terminator6/1  "Acceleration (Body)"
  Mux3/1 -> q_out/1, [q3]
  [q3dot] -> Gain2/1
  [C_hat3] -> Matrix Multiply3/1
  [g_hat3] -> Sum/3
  Matrix Multiply3/1 -> Sum/2
  Gain2/1 -> Add2/2
  Add/1 -> Add2/3  "r"
  Gain1/1 -> Add2/1
  MatrixMultiply/1 -> Sum/1
  Add2/1 -> Transpose1/1, MatrixMultiply/2
  [D_hat3] -> MatrixMultiply/1
  Demux1/5 -> Mux4/2
  [q3] -> Demux1/1
  Demux1/1 -> Terminator/1
  Demux1/6 -> Mux4/3
  Demux1/4 -> Mux4/1
  Mux4/1 -> eps_g/1(euler angles)
  Demux1/2 -> Terminator1/1
  Demux1/3 -> Terminator2/1
  Demux2/6 -> Mux5/3  "r"
  [q3dot] -> Demux2/1
  Demux2/4 -> Mux5/1  "p"
  Demux2/3 -> Terminator8/1
  Mux5/1 -> eps_c1_transpose/1(euler angles)
  Demux2/5 -> Mux5/2  "q"
  Demux2/2 -> Terminator7/1
  [q3] -> Mux6/1
  [q3dot] -> Transpose4/1, Mux6/2
  Mux6/1 -> Subtract/1
  Mux7/1 -> Subtract/2
  Gain/1 -> Multiply/1
  S/1 -> Gain/1
  Constant/1 -> Transpose/1
  Transpose/1 -> Multiply/2
  Multiply/1 -> Integrator/1
  Constant1/1 -> Multiply/3
  Subtract/1 -> Multiply/4, Multiply1/4  "e1"
  ref_q/1 -> Gain5/1, Mux7/1
  Transpose1/1 -> Multiply/5
  Transpose2/1 -> Multiply/6
  eps_d/1 -> Transpose2/1
  Integrator/1 -> MatrixMultiply1/1
  eps_d1/1 -> MatrixMultiply1/2
  MatrixMultiply1/1 -> [D_hat3]
  Transpose3/1 -> Multiply1/2
  S1/1 -> Gain3/1
  Gain3/1 -> Multiply1/1
  Constant2/1 -> Transpose3/1
  Constant4/1 -> Multiply1/3
  Multiply1/1 -> MatrixMultiply3/1, MatrixMultiply2/1
  Transpose4/1 -> MatrixMultiply2/2
  eps_c1_transpose/1(eps_c) -> Transpose6/1, MatrixMultiply2/3
  MatrixMultiply2/1 -> Integrator1/1
  Transpose5/1 -> MatrixMultiply3/2
  eps_g/1(eps_g) -> MatrixMultiply5/2, Transpose5/1
  Integrator1/1 -> MatrixMultiply4/1
  MatrixMultiply4/1 -> [C_hat3]
  MatrixMultiply3/1 -> Integrator2/1
  MatrixMultiply5/1 -> [g_hat3]
  Integrator2/1 -> MatrixMultiply5/1
  Transpose6/1 -> MatrixMultiply4/2

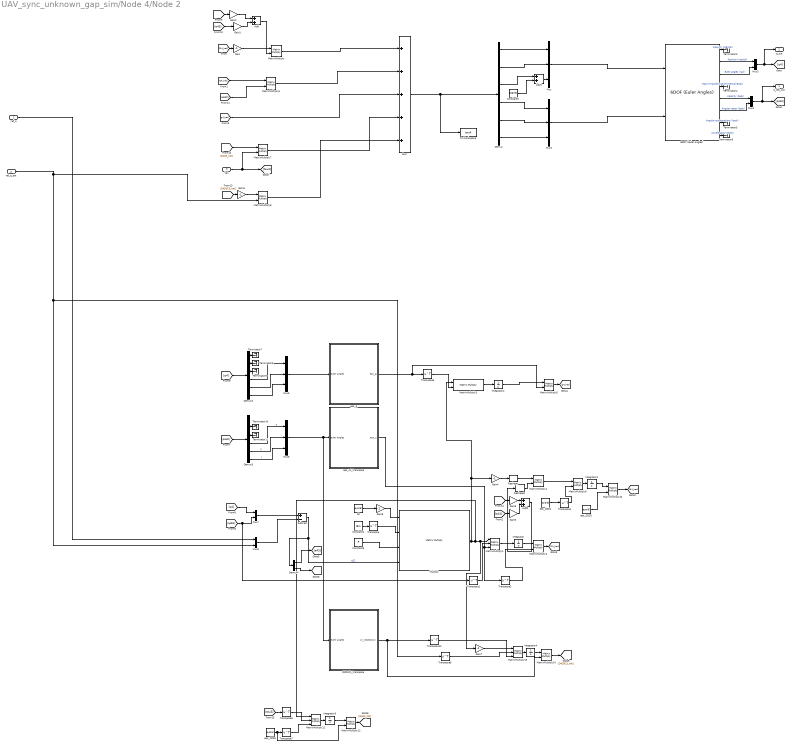
== system UAV_sync_unknown_gap_sim/Node 4/Node 2 ==
  ref_q : Inport
  ref_q_dot : Inport  Port=2
  tau : Inport  Port=3
  6DOF (Euler Angles) : shared6dof/6DOF (Euler Angles)  units=Metric (MKS)  mtype=Fixed  rep=Euler Angles  xme_0=init_pos4  Vm_0=init_vel4  eul_0=init_eul4  pm_0=init_ang4  mass_0=M4  mass_e=0.5  mass_f=2.0  inertia=I4  inertia_e=eye(3)  inertia_f=2*eye(3)  k_quat=1.0  vre_flag=on  abi_flag=off  aMode=aMode  xme_statename=''  Vm_statename=''  eul_statename=''  quat_statename=''  pm_statename=''  mass_statename=''
      settings: SourceProductBaseCode=AE
  Add : Sum
  Add1 : Sum
  Add2 : Sum
  Constant3 : Constant  Value=M4*G
  Constant4 : Constant  Value=Bm
  Constant5 : Constant  Value=P
  D2D1C1_transpose : Subsystem
  Demux : Demux  Outputs=6
  Demux2 : Demux  Outputs=6
  Demux3 : Demux  Outputs=6
  Demux4 : Demux  Outputs=2
  Gain{,3..4,7,9} (5 alike) : Gain  Gain=-1
  Gain1 : Gain  Gain=Kp  Multiplication=Matrix(K*u)
  Gain2 : Gain  Gain=Kv  Multiplication=Matrix(K*u)
  Gain5 : Gain  Gain=Kp  Multiplication=Matrix(K*u)
  Gain6 : Gain  Gain=Kv  Multiplication=Matrix(K*u)
  Integrator{,1..4} (5 alike) : Integrator
  MatrixMultiply{,2..10,12,14} (12 alike) : Product  Multiplication=Matrix(*)
  MatrixMultiply1 : Product  Inputs=3  Multiplication=Matrix(*)
  MatrixMultiply11 : Product  Inputs=3  Multiplication=Matrix(*)
  MatrixMultiply13 : Product  Inputs=3  Multiplication=Matrix(*)
  Multiply : Product  Inputs=4  Multiplication=Matrix(*)
  Mux{,1,5..6} (4 alike) : Mux  Inputs=3
  Mux{2..3,7..8} (4 alike) : Mux  Inputs=2
  Reshape : Reshape  OutputDimensionality=Column vector (2-D)
  Reshape1 : Reshape  OutputDimensionality=Row vector (2-D)
  S2 : Constant  Value=eye(6)
  Subtract : Sum  Inputs=+-
  Sum : Sum  Inputs=+++++
  Terminator{3..11} (9 alike) : Terminator
  To Workspace : ToWorkspace  VariableName=tau4  SaveFormat=Timeseries  SampleTime=-1
  Transpose{,1..2,4..8,10} (9 alike) : Math  Operator=transpose  SaturateOnIntegerOverflow=on
  eps_D2D1 : Constant  Value=eye(6)
  eps_D2D2 : Constant  Value=eye(6)
  eps_D2D3 : Constant  Value=eye(6)
  eps_c1_transpose : Subsystem
  eps_g : Subsystem
  q_dot_out : Outport
  q_out : Outport  Port=2
  wires:
  6DOF (Euler Angles)/3 -> Mux3/2  "Euler angles (rad)"
  6DOF (Euler Angles)/6 -> Mux2/2  "Angular rates (body)"
  6DOF (Euler Angles)/5 -> Mux2/1  "Velocity (body)"
  6DOF (Euler Angles)/2 -> Mux3/1  "Position (inertial)"
  ref_q/1 -> Mux8/1
  ref_q_dot/1 -> MatrixMultiply8/2, Transpose8/1, Mux8/2
  Sum/1 -> To Workspace/1, Demux/1
  Demux/1 -> Mux/1
  Demux/2 -> Mux/2
  Demux/6 -> Mux1/3
  Demux/5 -> Mux1/2
  Demux/4 -> Mux1/1
  Mux/1 -> 6DOF (Euler Angles)/1
  Mux1/1 -> 6DOF (Euler Angles)/2
  Mux2/1 -> q_dot_out/1, [q4dot]
  Add1/1 -> Mux/3
  Demux/3 -> Add1/1
  Constant3/1 -> Add1/2
  6DOF (Euler Angles)/1 -> Terminator3/1  "Velocity (inertial)"
  6DOF (Euler Angles)/4 -> Terminator4/1  "MatrixTransformation(Inertial-Body)"
  6DOF (Euler Angles)/7 -> Terminator5/1  "Angular accelerations (body)"
  6DOF (Euler Angles)/8 -> Terminator6/1  "Acceleration (Body)"
  Mux3/1 -> q_out/1, [q4]
  Demux2/6 -> Mux5/3
  Demux2/1 -> Terminator7/1
  Mux6/1 -> D2D1C1_transpose/1(euler angles), eps_c1_transpose/1(euler angles)
  Demux3/4 -> Mux6/1  "p"
  Demux3/6 -> Mux6/3  "r"
  Demux3/2 -> Terminator10/1
  Demux3/3 -> Terminator11/1
  Constant5/1 -> Multiply/3
  Subtract/1 -> Demux4/1, Multiply/4  "e21"
  Integrator2/1 -> MatrixMultiply5/1
  Demux2/5 -> Mux5/2
  MatrixMultiply10/1 -> [D4_hat]
  Demux3/5 -> Mux6/2  "q"
  Constant4/1 -> Transpose/1
  [q4] -> Mux7/1
  [q4dot] -> Transpose1/1, Mux7/2
  Transpose/1 -> Multiply/2
  S2/1 -> Gain9/1
  MatrixMultiply3/1 -> Integrator2/1
  MatrixMultiply5/1 -> [g4_hat]
  Mux5/1 -> eps_g/1(euler angles)
  Demux2/4 -> Mux5/1
  Demux2/3 -> Terminator9/1
  Demux2/2 -> Terminator8/1
  eps_c1_transpose/1(eps_c) -> Transpose2/1, MatrixMultiply1/3
  Gain9/1 -> Multiply/1
  Transpose5/1 -> MatrixMultiply3/2
  eps_g/1(eps_g) -> MatrixMultiply5/2, Transpose5/1
  [q4dot] -> Demux3/1
  [q4] -> Demux2/1
  Mux8/1 -> Subtract/2
  Mux7/1 -> Subtract/1
  [D4_hat] -> Gain/1
  Demux4/2 -> [e43_dot]
  Demux4/1 -> [e43]
  [e43] -> Gain1/1
  [e43_dot] -> Gain2/1
  Gain1/1 -> Add/2
  Gain2/1 -> Add/1
  Gain/1 -> MatrixMultiply/1
  Add/1 -> MatrixMultiply/2
  MatrixMultiply/1 -> Sum/1
  [C4_hat] -> MatrixMultiply6/1
  [q4dot] -> MatrixMultiply6/2
  MatrixMultiply6/1 -> Sum/2
  [g4_hat] -> Sum/3
  [D4D3_hat] -> MatrixMultiply7/1
  tau/1 -> [tau3], MatrixMultiply7/2
  MatrixMultiply7/1 -> Sum/4
  [D4D3C3_hat] -> Gain3/1
  Gain3/1 -> MatrixMultiply8/1
  MatrixMultiply8/1 -> Sum/5
  Transpose1/1 -> MatrixMultiply1/2
  MatrixMultiply2/1 -> [C4_hat]
  MatrixMultiply1/1 -> Integrator/1
  Transpose2/1 -> MatrixMultiply2/2
  Multiply/1 -> MatrixMultiply3/1, Gain4/1, MatrixMultiply11/1, Gain7/1, MatrixMultiply1/1
  Integrator/1 -> MatrixMultiply2/1
  [e43] -> Gain5/1
  [e43_dot] -> Gain6/1
  Gain6/1 -> Add2/1
  Gain5/1 -> Add2/2
  eps_D2D1/1 -> Transpose4/1
  MatrixMultiply4/1 -> MatrixMultiply9/1
  Transpose4/1 -> MatrixMultiply9/2
  MatrixMultiply9/1 -> Integrator1/1
  eps_D2D2/1 -> MatrixMultiply10/2
  [tau3] -> Transpose6/1
  Transpose6/1 -> MatrixMultiply11/2
  eps_D2D3/1 -> MatrixMultiply12/2, Transpose7/1
  Transpose7/1 -> MatrixMultiply11/3
  MatrixMultiply11/1 -> Integrator3/1
  Integrator3/1 -> MatrixMultiply12/1
  MatrixMultiply12/1 -> [D4D3_hat]
  Gain7/1 -> MatrixMultiply13/1
  Transpose8/1 -> MatrixMultiply13/2
  MatrixMultiply13/1 -> Integrator4/1
  Integrator4/1 -> MatrixMultiply14/1
  D2D1C1_transpose/1("\\xi_{D2D1C1}") -> MatrixMultiply14/2, Transpose10/1
  MatrixMultiply14/1 -> [D4D3C3_hat]
  Transpose10/1 -> MatrixMultiply13/3
  Integrator1/1 -> MatrixMultiply10/1
  Gain4/1 -> Reshape/1
  Add2/1 -> Reshape1/1
  Reshape1/1 -> MatrixMultiply4/2
  Reshape/1 -> MatrixMultiply4/1

== system UAV_sync_unknown_gap_sim/Node 0/Node 0/Derived Data ==
  note: WAE = Wind Angle Error
  In1 : Inport
  In2 : Inport  Port=2
  Bus Creator2 : BusCreator  Inputs=7
  Bus Selector : BusSelector  OutputSignals=WindVelocity(Body)
  Bus Selector5 : BusSelector  OutputSignals=Velocity (body),Velocity (inertial),Euler angles (rad)
  Constant9 : Constant  Value=C_rho
  Dynamic Pressure : aerolibasang/Dynamic Pressure
  "Incidence, Sideslip, & Airspeed" : aerolibasang/Incidence, Sideslip, & Airspeed
      settings: SourceProductName=Aerospace Blockset
  Scope : Scope
  Selector : Selector  InputPortWidth=3  IndexOptions=Index vector (dialog)  Indices=3  OutputSizes=1
  Selector1 : Selector  InputPortWidth=3  IndexOptions=Index vector (dialog)  Indices=2  OutputSizes=1
  Selector3 : Selector  InputPortWidth=3  IndexOptions=Index vector (dialog)  Indices=1  OutputSizes=1
  Sum2 : Sum  Inputs=|-+
  Sum4 : Sum  Inputs=+-|
  Sum5 : Sum  Inputs=+-|
  Trigonometric Function1 : Trigonometry  Operator=atan2
  Derived_Condition : Outport
  wires:
  In2/1 -> Bus Selector5/1
  "Incidence, Sideslip, & Airspeed"/2 -> Sum5/2, Bus Creator2/2  "beta"
  "Incidence, Sideslip, & Airspeed"/1 -> Bus Creator2/1  "alpha"
  Dynamic Pressure/1 -> Bus Creator2/4  "qbar"
  Sum2/1 -> "Incidence, Sideslip, & Airspeed"/1
  Constant9/1 -> Dynamic Pressure/2
  Bus Selector5/2 -> Selector1/1, Selector3/1  "<Velocity (inertial)>"
  Trigonometric Function1/1 -> Sum4/1, Bus Creator2/5  "course_angle"
  Bus Selector5/3 -> Selector/1  "<Euler angles (rad)>"
  Selector/1 -> Sum4/2
  Sum5/1 -> Bus Creator2/7  "WAE"
  "Incidence, Sideslip, & Airspeed"/3 -> Scope/1, Bus Creator2/3  "Va"
  Sum4/1 -> Sum5/1, Bus Creator2/6  "crab_angle"
  Bus Selector5/1 -> Dynamic Pressure/1, Sum2/2  "<Velocity (body)>"
  Bus Creator2/1 -> Derived_Condition/1
  In1/1 -> Bus Selector/1
  Bus Selector/1 -> Sum2/1  "<WindVelocity(Body)>"
  Selector1/1 -> Trigonometric Function1/1
  Selector3/1 -> Trigonometric Function1/2

== system UAV_sync_unknown_gap_sim/Node 0/Node 0/Inverse Dynamics Control ==
  References : Inport
  Aircraft Data : Inport  Port=2
  Constant8 : Constant  Value=g0
  Inverse Dynamic 1 : Subsystem
  Inverse Dynamic 2 : Subsystem
  D_qddot : Outport
  C_qdot : Outport  Port=2
  g(q) : Outport  Port=3
  wires:
  Inverse Dynamic 1/1(D_qddot) -> D_qddot/1
  References/1 -> Inverse Dynamic 1/1(References)
  Aircraft Data/1 -> Inverse Dynamic 2/1(Aricraft Data), Inverse Dynamic 1/2(Aircraft Data)
  Inverse Dynamic 2/1(C_qdot) -> C_qdot/1
  Constant8/1 -> g(q)/1

== system UAV_sync_unknown_gap_sim/Node 0/Node 0/Subsystem ==
  VF_System_Parameters : Inport
  Bus Creator1 : BusCreator  Inputs=18
  Demux : Demux  Outputs=18
  References : Outport
  wires:
  VF_System_Parameters/1 -> Demux/1
  Demux/7 -> Bus Creator1/7  "xdot_ref_final"
  Demux/6 -> Bus Creator1/6  "psi_ref_final"
  Demux/9 -> Bus Creator1/9  "hdot_ref_final"
  Demux/18 -> Bus Creator1/18  "psiddot_ref_final"
  Bus Creator1/1 -> References/1
  Demux/1 -> Bus Creator1/1  "x_ref _final"
  Demux/4 -> Bus Creator1/4  "phi_ref_final"
  Demux/5 -> Bus Creator1/5  "theta_ref_final"
  Demux/2 -> Bus Creator1/2  "y_ref_final"
  Demux/3 -> Bus Creator1/3  "h_ref_final"
  Demux/8 -> Bus Creator1/8  "ydot_ref_final"
  Demux/14 -> Bus Creator1/14  "yddot_ref_final"
  Demux/16 -> Bus Creator1/16  "phiddot_ref_final"
  Demux/15 -> Bus Creator1/15  "hddot_ref_final"
  Demux/10 -> Bus Creator1/10  "phidot_ref_final"
  Demux/13 -> Bus Creator1/13  "xddot_ref_final"
  Demux/17 -> Bus Creator1/17  "thetaddot_ref_final"
  Demux/12 -> Bus Creator1/12  "psidot_ref_final"
  Demux/11 -> Bus Creator1/11  "thetadot_ref_final"

== system UAV_sync_unknown_gap_sim/Node 0/Node 0/Wind ==
  In1 : Inport
  Bus Creator1 : BusCreator  Inputs=1
  Bus Selector4 : BusSelector  OutputSignals=MatrixTransformation(Inertial-Body)
  Constant1 : Constant  Value=InitWind
  Product : Product  Multiplication=Matrix(*)
  Out1 : Outport
  wires:
  Constant1/1 -> Product/2
  In1/1 -> Bus Selector4/1
  Bus Selector4/1 -> Product/1  "<MatrixTransformation(Inertial-Body)>"
  Product/1 -> Bus Creator1/1  "WindVelocity(Body)"
  Bus Creator1/1 -> Out1/1

== system UAV_sync_unknown_gap_sim/Node 0/VF Approach/AUTOPILOT ==
  note: In
  note: Out
  note: Autopilot controllers
      |
      | - Roll, pitch, side-slip control loops
      | - Total Energy Control System for the height and airspeed management
      | - Navigation controller for the course holding
  note: Sampling 400 Hz
  PlantData : Inport
  DerCond : Inport  Port=2
  EnvData : Inport  Port=3
  VF : Inport  Port=4
  GuidData : Inport  Port=5
  Bus Creator : BusCreator  Inputs=7
  Bus Creator1 : BusCreator  Inputs=3
  Bus Selector1 : BusSelector  OutputSignals=DerCond @400Hz
  Bus Selector2 : BusSelector  OutputSignals=chi_c_deg
  Bus Selector3 : BusSelector  OutputSignals=PlantData @400Hz
  Fly-by-wire inputs : Subsystem
  Goto Tag Visibility 1 : GotoTagVisibility  GotoTag=ThrottleDem
  Goto Tag Visibility 2 : GotoTagVisibility  GotoTag=RollDem
  Goto Tag Visibility 3 : GotoTagVisibility  GotoTag=PitchDem
  Ground : Ground
  Low-level Controllers : Subsystem
  Manual Switch4 : ManualSwitch  CurrentSetting=0
  Manual Switch9 : ManualSwitch
  Navigation Controller : Subsystem
  Scope : Scope
  Scope1 : Scope
  Step : Step  Time=10  Before=50  After=80  SampleTime=0
  Step1 : Step  Time=10  Before=15  After=20  SampleTime=0
  Target Airspeed : Constant  Value=Aero.AirspeedRef
  Target Height : Constant  Value=Aero.HeightRef
  Total Energy Control System : Subsystem
  Zero-Order Hold : ZeroOrderHold  SampleTime=1/400
  Zero-Order Hold1 : ZeroOrderHold  SampleTime=1/400
  Zero-Order Hold2 : ZeroOrderHold  SampleTime=1/400
  CtrBus. : Outport
  EnvData. : Outport  Port=2
  VF. : Outport  Port=3
  GuidData. : Outport  Port=4
  wires:
  Bus Creator1/1 -> [Reference]
  PlantData/1 -> Bus Selector3/1
  Low-level Controllers/4(RuddDemand) -> [rudder]
  Low-level Controllers/3(ElevDemand) -> [elevator]
  Low-level Controllers/2(AilDemand) -> Scope1/1, [ailerons]
  Low-level Controllers/1(ThrottOut) -> [throttle]
  [RollDem] -> Bus Creator1/2  "Roll Reference"
  [CourseRef] -> Navigation Controller/1(ReferenceCourse)
  [PlantData] -> Low-level Controllers/4(PlantData)
  Bus Selector1/1 -> [DerCond]  "<DerCond @400Hz>"
  DerCond/1 -> Bus Selector1/1
  [DerCond] -> Navigation Controller/2(DerCond)
  Bus Selector3/1 -> [PlantData]  "<PlantData @400Hz>"
  Manual Switch4/1 -> Zero-Order Hold1/1
  Manual Switch9/1 -> Zero-Order Hold2/1
  Step/1 -> Manual Switch4/1
  Target Height/1 -> Manual Switch4/2
  Target Airspeed/1 -> Manual Switch9/1
  Step1/1 -> Manual Switch9/2
  [PitchDem] -> Bus Creator1/1  "Pitch Reference"
  Zero-Order Hold/1 -> [CourseRef]
  [PlantData] -> Total Energy Control System/1(PlantData)
  EnvData/1 -> EnvData./1
  GuidData/1 -> GuidData./1
  VF/1 -> VF./1, Bus Selector2/1
  Bus Selector2/1 -> Zero-Order Hold/1  "<chi_c_deg>"
  [ThrottleDem] -> Bus Creator1/3  "Throttle Reference"
  Zero-Order Hold1/1 -> [Target_Height]
  Zero-Order Hold2/1 -> [Target_Airspeed]
  Total Energy Control System/1(ThrottleDem) -> Fly-by-wire inputs/1(Thr in)
  Total Energy Control System/2(PitchDem) -> Fly-by-wire inputs/2(Pitch in)
  Navigation Controller/1(BankAngle) -> Fly-by-wire inputs/4(Roll in)
  Fly-by-wire inputs/1(Thr out) -> Low-level Controllers/1(ThrottIn)
  Fly-by-wire inputs/2(Pitch out) -> Low-level Controllers/2(Pitch)
  Ground/1 -> Fly-by-wire inputs/3(.)
  [Target_Height] -> Total Energy Control System/2(Target_Height)
  [Target_Airspeed] -> Total Energy Control System/3(Target_Airspeed)
  [ailerons] -> Bus Creator/2  "ailerons"
  [throttle] -> Bus Creator/1  "throttle"
  [elevator] -> Bus Creator/3  "elevator"
  [rudder] -> Bus Creator/4  "rudder"
  [Reference] -> Bus Creator/5  "Out_references"
  [Target_Height] -> Bus Creator/6  "Target_height"
  [Target_Airspeed] -> Bus Creator/7  "Target_airspeed"
  Bus Creator/1 -> CtrBus./1
  Fly-by-wire inputs/3(Roll out) -> Low-level Controllers/3(Roll), Scope/1

== system UAV_sync_unknown_gap_sim/Node 0/VF Approach/BIXLER DYNAMICS ==
  note: This sub-block contains the dynamics of the aircraft.
      |
      | - All the states and quantities of interest are contained in the Bus signal PlantData.
      | - The derived conditions such as Airspeed, Angle of Attack, and Side-slip angle, are contained in Bus signal DerCond .
      | - The Bus EnvData contains the wind quantities of interest.
      | - The dynamical model is continuous, but the Buses are sampled to feed the discrete-time control system.
      | - The parameters of this block are contained in parameters/parameters_aero.
  ControlActions : Inport
  EnvData : Inport  Port=2
  GuidData : Inport  Port=3
  VF : Inport  Port=4
  Actuator Dynamics : Subsystem
  Bus Creator1 : BusCreator  Inputs='qbar','alpha','beta','Va','Course','CrabAngle','WAE'
  Bus Selector : BusSelector  OutputSignals=throttle
  Derived Conditions : Subsystem
  RUBBISH BIN : Subsystem
  Sampling : Subsystem
  "Sampling " : Subsystem
  Throttle Dynamics : Subsystem
  Vehicle Airframe : Subsystem
  PlantData. : Outport
  DerCond. : Outport  Port=2
  ControlBus. : Outport  Port=3
  GuidData. : Outport  Port=4
  VF. : Outport  Port=5
  wires:
  Bus Creator1/1 -> "Sampling "/1(Cont.), [DerCond]  "DerCond"
  Bus Selector/1 -> Throttle Dynamics/1(In)  "<throttle>"
  Throttle Dynamics/1(Out) -> Vehicle Airframe/1(Throttle_cmd)  "throttle"
  ControlActions/1 -> ControlBus./1, Bus Selector/1, Actuator Dynamics/1(In)
  Actuator Dynamics/1(Out) -> Vehicle Airframe/2(ControlActions)
  Vehicle Airframe/1(PlantData) -> [PlantData], Sampling/1(Cont.)  "PlantData"
  Sampling/1(Cont.+Disc.) -> PlantData./1
  "Sampling "/1(Cont.+Disc.) -> DerCond./1
  GuidData/1 -> GuidData./1
  VF/1 -> VF./1
  [PlantData] -> Derived Conditions/2(PlantData)
  EnvData/1 -> Derived Conditions/1(EnvData)
  Derived Conditions/1(qbar) -> Bus Creator1/1  "qbar"
  Derived Conditions/2(alpha) -> Bus Creator1/2  "alpha"
  Derived Conditions/4(Va) -> Bus Creator1/4  "Va"
  Derived Conditions/3(beta) -> Bus Creator1/3  "beta"
  Derived Conditions/5(CourseAngle) -> Bus Creator1/5  "Course"
  Derived Conditions/6(CrabAngle) -> Bus Creator1/6  "CrabAngle"
  Derived Conditions/7(WAE) -> Bus Creator1/7  "WAE"
  [DerCond] -> Vehicle Airframe/3(DerCond)
